simulink model "While_Counter"  (R2017b)
settings: Solver=FixedStepDiscrete  StartTime=0.0  StopTime=10.0  RelTol=1e-3
settings Model: Creator=engdo  LastModifiedBy=engdo
settings OptimizationCC: DefaultParameterBehavior=Inlined  PassReuseOutputArgsAs=Individual arguments
settings DebuggingCC: ParameterTunabilityLossMsg=error
settings SFSimCC: MATLABDynamicMemAlloc=off
settings RTWCC: SystemTargetFile=ert.tlc  GenCodeOnly=on  TemplateMakefile=ert_default_tmf  GenerateReport=on  IncludeHyperlinkInReport=on  LaunchReport=on  GenerateTraceInfo=on  GenerateTraceReport=on  GenerateTraceReportSl=on  GenerateTraceReportSf=on  GenerateTraceReportEml=on  GenerateWebview=on
settings CodeAppCC: ForceParamTrailComments=on  IgnoreCustomStorageClasses=off  OperatorAnnotations=on  SimulinkDataObjDesc=on  SFDataObjDesc=on  InsertBlockDesc=on
settings ERTTargetCC: TargetLangStandard=C99 (ISO)  GenerateSampleERTMain=on  InlinedParameterPlacement=NonHierarchical  ERTCustomFileTemplate=example_file_process.tlc  EnableUserReplacementTypes=on

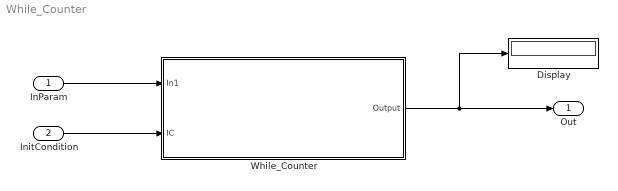
== system While_Counter ==
  InParam : Inport
  InitCondition : Inport  Port=2
  Display : Display
  While_Counter : Subsystem  TreatAsAtomicUnit=on
  Out : Outport
  wires:
  InParam/1 -> While_Counter/1(In1)
  InitCondition/1 -> While_Counter/2(IC)
  While_Counter/1(Output) -> Display/1, Out/1

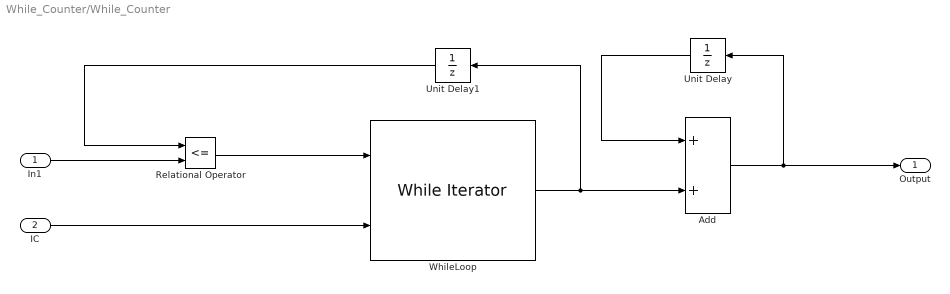
== system While_Counter/While_Counter ==
  In1 : Inport
  IC : Inport  Port=2
  Add : Sum
  Relational Operator : RelationalOperator  Operator=<=  OutDataTypeStr=boolean  RndMeth=Simplest
  Unit Delay : UnitDelay  SampleTime=-1
  Unit Delay1 : UnitDelay  SampleTime=-1
  WhileLoop : WhileIterator  ShowIterationPort=on
  Output : Outport
  wires:
  IC/1 -> WhileLoop/2
  Add/1 -> Output/1, Unit Delay/1
  Unit Delay1/1 -> Relational Operator/1
  Relational Operator/1 -> WhileLoop/1
  In1/1 -> Relational Operator/2
  WhileLoop/1 -> Unit Delay1/1, Add/2
  Unit Delay/1 -> Add/1
